simulink model "przyklad_mateusz"  (R2023a)
settings: Solver=ode1  StartTime=0.0  StopTime=inf  FixedStep=0.0001  RelTol=1e-3  EnableMultiTasking=on
undefined symbols (not defined in the file): DiscIntNeverNeededParam, sigbuilder_block
libraries: stm32f4xxblockslib x8, simulink x7, stm32blockslib x6, stmutilitieslib x3, stm32f7xxblockslib x3
(part 2 of 2)

== system przyklad_mateusz/obiekt/fuzzy/Fuzzy Type 2/nbM5 ==
  x : Inport
  Add : Sum  Inputs=+-
  Add1 : Sum  Inputs=-+
  Add2 : Sum  Inputs=+-
  Add3 : Sum  Inputs=-+
  Constant : Constant
  Constant1 : Constant
  Constant2 : Constant  Value=0
  Divide : Product  Inputs=*/
  Divide1 : Product  Inputs=*/
  Max : MinMax  Function=max  Inputs=2
  Min : MinMax  Inputs=2
  Switch : Switch  Criteria=u2 > Threshold  SaturateOnIntegerOverflow=off  InputSameDT=off
  Switch1 : Switch  Criteria=u2 > Threshold  SaturateOnIntegerOverflow=off  InputSameDT=off
  a : Constant  Value=-1.8
  b : Constant  Value=-1
  c : Constant  Value=-0.2
  Out1 : Outport
  wires:
  x/1 -> Add2/2, Add/1
  a/1 -> Add1/1, Add/2
  b/1 -> Add1/2, Add3/1
  c/1 -> Add2/1, Add3/2
  Add/1 -> Divide/1
  Divide1/1 -> Switch1/1
  Divide/1 -> Switch/1
  Add1/1 -> Switch/2, Divide/2
  Add2/1 -> Divide1/1
  Add3/1 -> Switch1/2, Divide1/2
  Constant/1 -> Switch/3
  Constant1/1 -> Switch1/3
  Switch/1 -> Min/1
  Switch1/1 -> Min/2
  Min/1 -> Max/2
  Constant2/1 -> Max/1
  Max/1 -> Out1/1

== system przyklad_mateusz/obiekt/fuzzy/Fuzzy Type 2/pbM2 ==
  x : Inport
  Add : Sum  Inputs=+-
  Add1 : Sum  Inputs=-+
  Add2 : Sum  Inputs=+-
  Add3 : Sum  Inputs=-+
  Constant : Constant
  Constant1 : Constant
  Constant2 : Constant  Value=0
  Divide : Product  Inputs=*/
  Divide1 : Product  Inputs=*/
  Max : MinMax  Function=max  Inputs=2
  Min : MinMax  Inputs=2
  Switch : Switch  Criteria=u2 > Threshold  SaturateOnIntegerOverflow=off  InputSameDT=off
  Switch1 : Switch  Criteria=u2 > Threshold  SaturateOnIntegerOverflow=off  InputSameDT=off
  a : Constant  Value=0
  b : Constant
  c : Constant  Value=2
  Out1 : Outport
  wires:
  Max/1 -> Out1/1
  Constant2/1 -> Max/1
  Min/1 -> Max/2
  Switch1/1 -> Min/2
  Switch/1 -> Min/1
  Constant1/1 -> Switch1/3
  Constant/1 -> Switch/3
  Add3/1 -> Divide1/2, Switch1/2
  Add2/1 -> Divide1/1
  Add1/1 -> Divide/2, Switch/2
  Divide/1 -> Switch/1
  Divide1/1 -> Switch1/1
  Add/1 -> Divide/1
  c/1 -> Add3/2, Add2/1
  b/1 -> Add3/1, Add1/2
  a/1 -> Add/2, Add1/1
  x/1 -> Add/1, Add2/2

== system przyklad_mateusz/obiekt/fuzzy/Fuzzy Type 2/pbM3 ==
  x : Inport
  Add : Sum  Inputs=+-
  Add1 : Sum  Inputs=-+
  Add2 : Sum  Inputs=+-
  Add3 : Sum  Inputs=-+
  Constant : Constant
  Constant1 : Constant
  Constant2 : Constant  Value=0
  Divide : Product  Inputs=*/
  Divide1 : Product  Inputs=*/
  Max : MinMax  Function=max  Inputs=2
  Min : MinMax  Inputs=2
  Switch : Switch  Criteria=u2 > Threshold  SaturateOnIntegerOverflow=off  InputSameDT=off
  Switch1 : Switch  Criteria=u2 > Threshold  SaturateOnIntegerOverflow=off  InputSameDT=off
  a : Constant  Value=0
  b : Constant
  c : Constant  Value=2
  Out1 : Outport
  wires:
  Max/1 -> Out1/1
  Constant2/1 -> Max/1
  Min/1 -> Max/2
  Switch1/1 -> Min/2
  Switch/1 -> Min/1
  Constant1/1 -> Switch1/3
  Constant/1 -> Switch/3
  Add3/1 -> Divide1/2, Switch1/2
  Add2/1 -> Divide1/1
  Add1/1 -> Divide/2, Switch/2
  Divide/1 -> Switch/1
  Divide1/1 -> Switch1/1
  Add/1 -> Divide/1
  c/1 -> Add3/2, Add2/1
  b/1 -> Add3/1, Add1/2
  a/1 -> Add/2, Add1/1
  x/1 -> Add/1, Add2/2

== system przyklad_mateusz/obiekt/fuzzy/Fuzzy Type 2/pbM4 ==
  x : Inport
  Add : Sum  Inputs=+-
  Add1 : Sum  Inputs=-+
  Add2 : Sum  Inputs=+-
  Add3 : Sum  Inputs=-+
  Constant : Constant
  Constant1 : Constant
  Constant2 : Constant  Value=0
  Divide : Product  Inputs=*/
  Divide1 : Product  Inputs=*/
  Max : MinMax  Function=max  Inputs=2
  Min : MinMax  Inputs=2
  Switch : Switch  Criteria=u2 > Threshold  SaturateOnIntegerOverflow=off  InputSameDT=off
  Switch1 : Switch  Criteria=u2 > Threshold  SaturateOnIntegerOverflow=off  InputSameDT=off
  a : Constant  Value=0.2
  b : Constant
  c : Constant  Value=1.8
  Out1 : Outport
  wires:
  x/1 -> Add2/2, Add/1
  a/1 -> Add1/1, Add/2
  b/1 -> Add1/2, Add3/1
  c/1 -> Add2/1, Add3/2
  Add/1 -> Divide/1
  Divide1/1 -> Switch1/1
  Divide/1 -> Switch/1
  Add1/1 -> Switch/2, Divide/2
  Add2/1 -> Divide1/1
  Add3/1 -> Switch1/2, Divide1/2
  Constant/1 -> Switch/3
  Constant1/1 -> Switch1/3
  Switch/1 -> Min/1
  Switch1/1 -> Min/2
  Min/1 -> Max/2
  Constant2/1 -> Max/1
  Max/1 -> Out1/1

== system przyklad_mateusz/obiekt/fuzzy/Fuzzy Type 2/pbM5 ==
  x : Inport
  Add : Sum  Inputs=+-
  Add1 : Sum  Inputs=-+
  Add2 : Sum  Inputs=+-
  Add3 : Sum  Inputs=-+
  Constant : Constant
  Constant1 : Constant
  Constant2 : Constant  Value=0
  Divide : Product  Inputs=*/
  Divide1 : Product  Inputs=*/
  Max : MinMax  Function=max  Inputs=2
  Min : MinMax  Inputs=2
  Switch : Switch  Criteria=u2 > Threshold  SaturateOnIntegerOverflow=off  InputSameDT=off
  Switch1 : Switch  Criteria=u2 > Threshold  SaturateOnIntegerOverflow=off  InputSameDT=off
  a : Constant  Value=0.2
  b : Constant
  c : Constant  Value=1.8
  Out1 : Outport
  wires:
  x/1 -> Add2/2, Add/1
  a/1 -> Add1/1, Add/2
  b/1 -> Add1/2, Add3/1
  c/1 -> Add2/1, Add3/2
  Add/1 -> Divide/1
  Divide1/1 -> Switch1/1
  Divide/1 -> Switch/1
  Add1/1 -> Switch/2, Divide/2
  Add2/1 -> Divide1/1
  Add3/1 -> Switch1/2, Divide1/2
  Constant/1 -> Switch/3
  Constant1/1 -> Switch1/3
  Switch/1 -> Min/1
  Switch1/1 -> Min/2
  Min/1 -> Max/2
  Constant2/1 -> Max/1
  Max/1 -> Out1/1

== system przyklad_mateusz/obiekt/fuzzy/Fuzzy Type 2/zeM2 ==
  x : Inport
  Add : Sum  Inputs=+-
  Add1 : Sum  Inputs=-+
  Add2 : Sum  Inputs=+-
  Add3 : Sum  Inputs=-+
  Constant : Constant
  Constant1 : Constant
  Constant2 : Constant  Value=0
  Divide : Product  Inputs=*/
  Divide1 : Product  Inputs=*/
  Max : MinMax  Function=max  Inputs=2
  Min : MinMax  Inputs=2
  Switch : Switch  Criteria=u2 > Threshold  SaturateOnIntegerOverflow=off  InputSameDT=off
  Switch1 : Switch  Criteria=u2 > Threshold  SaturateOnIntegerOverflow=off  InputSameDT=off
  a : Constant  Value=-1
  b : Constant  Value=0
  c : Constant
  Out1 : Outport
  wires:
  Max/1 -> Out1/1
  Constant2/1 -> Max/1
  Min/1 -> Max/2
  Switch1/1 -> Min/2
  Switch/1 -> Min/1
  Constant1/1 -> Switch1/3
  Constant/1 -> Switch/3
  Add3/1 -> Divide1/2, Switch1/2
  Add2/1 -> Divide1/1
  Add1/1 -> Divide/2, Switch/2
  Divide/1 -> Switch/1
  Divide1/1 -> Switch1/1
  Add/1 -> Divide/1
  c/1 -> Add3/2, Add2/1
  b/1 -> Add3/1, Add1/2
  a/1 -> Add/2, Add1/1
  x/1 -> Add/1, Add2/2

== system przyklad_mateusz/obiekt/fuzzy/Fuzzy Type 2/zeM3 ==
  x : Inport
  Add : Sum  Inputs=+-
  Add1 : Sum  Inputs=-+
  Add2 : Sum  Inputs=+-
  Add3 : Sum  Inputs=-+
  Constant : Constant
  Constant1 : Constant
  Constant2 : Constant  Value=0
  Divide : Product  Inputs=*/
  Divide1 : Product  Inputs=*/
  Max : MinMax  Function=max  Inputs=2
  Min : MinMax  Inputs=2
  Switch : Switch  Criteria=u2 > Threshold  SaturateOnIntegerOverflow=off  InputSameDT=off
  Switch1 : Switch  Criteria=u2 > Threshold  SaturateOnIntegerOverflow=off  InputSameDT=off
  a : Constant  Value=-1
  b : Constant  Value=0
  c : Constant
  Out1 : Outport
  wires:
  Max/1 -> Out1/1
  Constant2/1 -> Max/1
  Min/1 -> Max/2
  Switch1/1 -> Min/2
  Switch/1 -> Min/1
  Constant1/1 -> Switch1/3
  Constant/1 -> Switch/3
  Add3/1 -> Divide1/2, Switch1/2
  Add2/1 -> Divide1/1
  Add1/1 -> Divide/2, Switch/2
  Divide/1 -> Switch/1
  Divide1/1 -> Switch1/1
  Add/1 -> Divide/1
  c/1 -> Add3/2, Add2/1
  b/1 -> Add3/1, Add1/2
  a/1 -> Add/2, Add1/1
  x/1 -> Add/1, Add2/2

== system przyklad_mateusz/obiekt/fuzzy/Fuzzy Type 2/zeM4 ==
  x : Inport
  Add : Sum  Inputs=+-
  Add1 : Sum  Inputs=-+
  Add2 : Sum  Inputs=+-
  Add3 : Sum  Inputs=-+
  Constant : Constant
  Constant1 : Constant
  Constant2 : Constant  Value=0
  Divide : Product  Inputs=*/
  Divide1 : Product  Inputs=*/
  Max : MinMax  Function=max  Inputs=2
  Min : MinMax  Inputs=2
  Switch : Switch  Criteria=u2 > Threshold  SaturateOnIntegerOverflow=off  InputSameDT=off
  Switch1 : Switch  Criteria=u2 > Threshold  SaturateOnIntegerOverflow=off  InputSameDT=off
  a : Constant  Value=-0.8
  b : Constant  Value=0
  c : Constant  Value=0.8
  Out1 : Outport
  wires:
  x/1 -> Add2/2, Add/1
  a/1 -> Add1/1, Add/2
  b/1 -> Add1/2, Add3/1
  c/1 -> Add2/1, Add3/2
  Add/1 -> Divide/1
  Divide1/1 -> Switch1/1
  Divide/1 -> Switch/1
  Add1/1 -> Switch/2, Divide/2
  Add2/1 -> Divide1/1
  Add3/1 -> Switch1/2, Divide1/2
  Constant/1 -> Switch/3
  Constant1/1 -> Switch1/3
  Switch/1 -> Min/1
  Switch1/1 -> Min/2
  Min/1 -> Max/2
  Constant2/1 -> Max/1
  Max/1 -> Out1/1

== system przyklad_mateusz/obiekt/fuzzy/Fuzzy Type 2/zeM5 ==
  x : Inport
  Add : Sum  Inputs=+-
  Add1 : Sum  Inputs=-+
  Add2 : Sum  Inputs=+-
  Add3 : Sum  Inputs=-+
  Constant : Constant
  Constant1 : Constant
  Constant2 : Constant  Value=0
  Divide : Product  Inputs=*/
  Divide1 : Product  Inputs=*/
  Max : MinMax  Function=max  Inputs=2
  Min : MinMax  Inputs=2
  Switch : Switch  Criteria=u2 > Threshold  SaturateOnIntegerOverflow=off  InputSameDT=off
  Switch1 : Switch  Criteria=u2 > Threshold  SaturateOnIntegerOverflow=off  InputSameDT=off
  a : Constant  Value=-0.8
  b : Constant  Value=0
  c : Constant  Value=0.8
  Out1 : Outport
  wires:
  x/1 -> Add2/2, Add/1
  a/1 -> Add1/1, Add/2
  b/1 -> Add1/2, Add3/1
  c/1 -> Add2/1, Add3/2
  Add/1 -> Divide/1
  Divide1/1 -> Switch1/1
  Divide/1 -> Switch/1
  Add1/1 -> Switch/2, Divide/2
  Add2/1 -> Divide1/1
  Add3/1 -> Switch1/2, Divide1/2
  Constant/1 -> Switch/3
  Constant1/1 -> Switch1/3
  Switch/1 -> Min/1
  Switch1/1 -> Min/2
  Min/1 -> Max/2
  Constant2/1 -> Max/1
  Max/1 -> Out1/1

== system przyklad_mateusz/Subsystem1/Subsystem/Enkoder/zliczanie enkodera/If Action Subsystem ==
  Input : Inport
  Input2 : Inport  Port=2
  Action Port : ActionPort
  If : If  IfExpression=u1 == 0  ShowElse=off
  If Action Subsystem : Subsystem  TreatAsAtomicUnit=on
  Out1 : Outport
  wires:
  Input/1 -> If/1
  If/1 -> If Action Subsystem/Action
  Input2/1 -> If Action Subsystem/1(Input2)
  If Action Subsystem/1(Out1) -> Out1/1

== system przyklad_mateusz/Subsystem1/Subsystem/Enkoder/zliczanie enkodera/If Action Subsystem2 ==
  Input : Inport
  Input2 : Inport  Port=2
  Action Port : ActionPort
  If : If  IfExpression=u1 == 1  ShowElse=off
  If Action Subsystem : Subsystem  TreatAsAtomicUnit=on
  Out1 : Outport
  wires:
  If Action Subsystem/1(Out1) -> Out1/1
  Input2/1 -> If Action Subsystem/1(Input2)
  If/1 -> If Action Subsystem/Action
  Input/1 -> If/1

== system przyklad_mateusz/Subsystem1/Subsystem/Obiekt/Moj/nbM ==
  x : Inport
  Add : Sum  Inputs=+-
  Add1 : Sum  Inputs=-+
  Add2 : Sum  Inputs=+-
  Add3 : Sum  Inputs=-+
  Constant : Constant
  Constant1 : Constant
  Constant2 : Constant  Value=0
  Divide : Product  Inputs=*/
  Divide1 : Product  Inputs=*/
  Max : MinMax  Function=max  Inputs=2
  Min : MinMax  Inputs=2
  Switch : Switch  Criteria=u2 > Threshold  SaturateOnIntegerOverflow=off  InputSameDT=off
  Switch1 : Switch  Criteria=u2 > Threshold  SaturateOnIntegerOverflow=off  InputSameDT=off
  a : Constant  Value=-2
  b : Constant  Value=-1
  c : Constant  Value=0
  Out1 : Outport
  wires:
  x/1 -> Add2/2, Add/1
  a/1 -> Add1/1, Add/2
  b/1 -> Add1/2, Add3/1
  c/1 -> Add2/1, Add3/2
  Add/1 -> Divide/1
  Divide1/1 -> Switch1/1
  Divide/1 -> Switch/1
  Add1/1 -> Switch/2, Divide/2
  Add2/1 -> Divide1/1
  Add3/1 -> Switch1/2, Divide1/2
  Constant/1 -> Switch/3
  Constant1/1 -> Switch1/3
  Switch/1 -> Min/1
  Switch1/1 -> Min/2
  Min/1 -> Max/2
  Constant2/1 -> Max/1
  Max/1 -> Out1/1

== system przyklad_mateusz/Subsystem1/Subsystem/Obiekt/Moj/nbM1 ==
  x : Inport
  Add : Sum  Inputs=+-
  Add1 : Sum  Inputs=-+
  Add2 : Sum  Inputs=+-
  Add3 : Sum  Inputs=-+
  Constant : Constant
  Constant1 : Constant
  Constant2 : Constant  Value=0
  Divide : Product  Inputs=*/
  Divide1 : Product  Inputs=*/
  Max : MinMax  Function=max  Inputs=2
  Min : MinMax  Inputs=2
  Switch : Switch  Criteria=u2 > Threshold  SaturateOnIntegerOverflow=off  InputSameDT=off
  Switch1 : Switch  Criteria=u2 > Threshold  SaturateOnIntegerOverflow=off  InputSameDT=off
  a : Constant  Value=-2
  b : Constant  Value=-1
  c : Constant  Value=0
  Out1 : Outport
  wires:
  x/1 -> Add2/2, Add/1
  a/1 -> Add1/1, Add/2
  b/1 -> Add1/2, Add3/1
  c/1 -> Add2/1, Add3/2
  Add/1 -> Divide/1
  Divide1/1 -> Switch1/1
  Divide/1 -> Switch/1
  Add1/1 -> Switch/2, Divide/2
  Add2/1 -> Divide1/1
  Add3/1 -> Switch1/2, Divide1/2
  Constant/1 -> Switch/3
  Constant1/1 -> Switch1/3
  Switch/1 -> Min/1
  Switch1/1 -> Min/2
  Min/1 -> Max/2
  Constant2/1 -> Max/1
  Max/1 -> Out1/1

== system przyklad_mateusz/Subsystem1/Subsystem/Obiekt/Moj/pbM ==
  x : Inport
  Add : Sum  Inputs=+-
  Add1 : Sum  Inputs=-+
  Add2 : Sum  Inputs=+-
  Add3 : Sum  Inputs=-+
  Constant : Constant
  Constant1 : Constant
  Constant2 : Constant  Value=0
  Divide : Product  Inputs=*/
  Divide1 : Product  Inputs=*/
  Max : MinMax  Function=max  Inputs=2
  Min : MinMax  Inputs=2
  Switch : Switch  Criteria=u2 > Threshold  SaturateOnIntegerOverflow=off  InputSameDT=off
  Switch1 : Switch  Criteria=u2 > Threshold  SaturateOnIntegerOverflow=off  InputSameDT=off
  a : Constant  Value=0
  b : Constant
  c : Constant  Value=2
  Out1 : Outport
  wires:
  x/1 -> Add2/2, Add/1
  a/1 -> Add1/1, Add/2
  b/1 -> Add1/2, Add3/1
  c/1 -> Add2/1, Add3/2
  Add/1 -> Divide/1
  Divide1/1 -> Switch1/1
  Divide/1 -> Switch/1
  Add1/1 -> Switch/2, Divide/2
  Add2/1 -> Divide1/1
  Add3/1 -> Switch1/2, Divide1/2
  Constant/1 -> Switch/3
  Constant1/1 -> Switch1/3
  Switch/1 -> Min/1
  Switch1/1 -> Min/2
  Min/1 -> Max/2
  Constant2/1 -> Max/1
  Max/1 -> Out1/1

== system przyklad_mateusz/Subsystem1/Subsystem/Obiekt/Moj/pbM1 ==
  x : Inport
  Add : Sum  Inputs=+-
  Add1 : Sum  Inputs=-+
  Add2 : Sum  Inputs=+-
  Add3 : Sum  Inputs=-+
  Constant : Constant
  Constant1 : Constant
  Constant2 : Constant  Value=0
  Divide : Product  Inputs=*/
  Divide1 : Product  Inputs=*/
  Max : MinMax  Function=max  Inputs=2
  Min : MinMax  Inputs=2
  Switch : Switch  Criteria=u2 > Threshold  SaturateOnIntegerOverflow=off  InputSameDT=off
  Switch1 : Switch  Criteria=u2 > Threshold  SaturateOnIntegerOverflow=off  InputSameDT=off
  a : Constant  Value=0
  b : Constant
  c : Constant  Value=2
  Out1 : Outport
  wires:
  x/1 -> Add2/2, Add/1
  a/1 -> Add1/1, Add/2
  b/1 -> Add1/2, Add3/1
  c/1 -> Add2/1, Add3/2
  Add/1 -> Divide/1
  Divide1/1 -> Switch1/1
  Divide/1 -> Switch/1
  Add1/1 -> Switch/2, Divide/2
  Add2/1 -> Divide1/1
  Add3/1 -> Switch1/2, Divide1/2
  Constant/1 -> Switch/3
  Constant1/1 -> Switch1/3
  Switch/1 -> Min/1
  Switch1/1 -> Min/2
  Min/1 -> Max/2
  Constant2/1 -> Max/1
  Max/1 -> Out1/1

== system przyklad_mateusz/Subsystem1/Subsystem/Obiekt/Moj/zeM ==
  x : Inport
  Add : Sum  Inputs=+-
  Add1 : Sum  Inputs=-+
  Add2 : Sum  Inputs=+-
  Add3 : Sum  Inputs=-+
  Constant : Constant
  Constant1 : Constant
  Constant2 : Constant  Value=0
  Divide : Product  Inputs=*/
  Divide1 : Product  Inputs=*/
  Max : MinMax  Function=max  Inputs=2
  Min : MinMax  Inputs=2
  Switch : Switch  Criteria=u2 > Threshold  SaturateOnIntegerOverflow=off  InputSameDT=off
  Switch1 : Switch  Criteria=u2 > Threshold  SaturateOnIntegerOverflow=off  InputSameDT=off
  a : Constant  Value=-1
  b : Constant  Value=0
  c : Constant
  Out1 : Outport
  wires:
  x/1 -> Add2/2, Add/1
  a/1 -> Add1/1, Add/2
  b/1 -> Add1/2, Add3/1
  c/1 -> Add2/1, Add3/2
  Add/1 -> Divide/1
  Divide1/1 -> Switch1/1
  Divide/1 -> Switch/1
  Add1/1 -> Switch/2, Divide/2
  Add2/1 -> Divide1/1
  Add3/1 -> Switch1/2, Divide1/2
  Constant/1 -> Switch/3
  Constant1/1 -> Switch1/3
  Switch/1 -> Min/1
  Switch1/1 -> Min/2
  Min/1 -> Max/2
  Constant2/1 -> Max/1
  Max/1 -> Out1/1

== system przyklad_mateusz/Subsystem1/Subsystem/Obiekt/Moj/zeM1 ==
  x : Inport
  Add : Sum  Inputs=+-
  Add1 : Sum  Inputs=-+
  Add2 : Sum  Inputs=+-
  Add3 : Sum  Inputs=-+
  Constant : Constant
  Constant1 : Constant
  Constant2 : Constant  Value=0
  Divide : Product  Inputs=*/
  Divide1 : Product  Inputs=*/
  Max : MinMax  Function=max  Inputs=2
  Min : MinMax  Inputs=2
  Switch : Switch  Criteria=u2 > Threshold  SaturateOnIntegerOverflow=off  InputSameDT=off
  Switch1 : Switch  Criteria=u2 > Threshold  SaturateOnIntegerOverflow=off  InputSameDT=off
  a : Constant  Value=-1
  b : Constant  Value=0
  c : Constant
  Out1 : Outport
  wires:
  x/1 -> Add2/2, Add/1
  a/1 -> Add1/1, Add/2
  b/1 -> Add1/2, Add3/1
  c/1 -> Add2/1, Add3/2
  Add/1 -> Divide/1
  Divide1/1 -> Switch1/1
  Divide/1 -> Switch/1
  Add1/1 -> Switch/2, Divide/2
  Add2/1 -> Divide1/1
  Add3/1 -> Switch1/2, Divide1/2
  Constant/1 -> Switch/3
  Constant1/1 -> Switch1/3
  Switch/1 -> Min/1
  Switch1/1 -> Min/2
  Min/1 -> Max/2
  Constant2/1 -> Max/1
  Max/1 -> Out1/1

== system przyklad_mateusz/Subsystem1/Subsystem/regulator/fuzzy/nbM ==
  x : Inport
  Add : Sum  Inputs=+-
  Add1 : Sum  Inputs=-+
  Add2 : Sum  Inputs=+-
  Add3 : Sum  Inputs=-+
  Constant : Constant
  Constant1 : Constant
  Constant2 : Constant  Value=0
  Divide : Product  Inputs=*/
  Divide1 : Product  Inputs=*/
  Max : MinMax  Function=max  Inputs=2
  Min : MinMax  Inputs=2
  Switch : Switch  Criteria=u2 > Threshold  SaturateOnIntegerOverflow=off  InputSameDT=off
  Switch1 : Switch  Criteria=u2 > Threshold  SaturateOnIntegerOverflow=off  InputSameDT=off
  a : Constant  Value=-2
  b : Constant  Value=-1
  c : Constant  Value=0
  Out1 : Outport
  wires:
  x/1 -> Add2/2, Add/1
  a/1 -> Add1/1, Add/2
  b/1 -> Add1/2, Add3/1
  c/1 -> Add2/1, Add3/2
  Add/1 -> Divide/1
  Divide1/1 -> Switch1/1
  Divide/1 -> Switch/1
  Add1/1 -> Switch/2, Divide/2
  Add2/1 -> Divide1/1
  Add3/1 -> Switch1/2, Divide1/2
  Constant/1 -> Switch/3
  Constant1/1 -> Switch1/3
  Switch/1 -> Min/1
  Switch1/1 -> Min/2
  Min/1 -> Max/2
  Constant2/1 -> Max/1
  Max/1 -> Out1/1

== system przyklad_mateusz/Subsystem1/Subsystem/regulator/fuzzy/nbM1 ==
  x : Inport
  Add : Sum  Inputs=+-
  Add1 : Sum  Inputs=-+
  Add2 : Sum  Inputs=+-
  Add3 : Sum  Inputs=-+
  Constant : Constant
  Constant1 : Constant
  Constant2 : Constant  Value=0
  Divide : Product  Inputs=*/
  Divide1 : Product  Inputs=*/
  Max : MinMax  Function=max  Inputs=2
  Min : MinMax  Inputs=2
  Switch : Switch  Criteria=u2 > Threshold  SaturateOnIntegerOverflow=off  InputSameDT=off
  Switch1 : Switch  Criteria=u2 > Threshold  SaturateOnIntegerOverflow=off  InputSameDT=off
  a : Constant  Value=-2
  b : Constant  Value=-1
  c : Constant  Value=0
  Out1 : Outport
  wires:
  x/1 -> Add2/2, Add/1
  a/1 -> Add1/1, Add/2
  b/1 -> Add1/2, Add3/1
  c/1 -> Add2/1, Add3/2
  Add/1 -> Divide/1
  Divide1/1 -> Switch1/1
  Divide/1 -> Switch/1
  Add1/1 -> Switch/2, Divide/2
  Add2/1 -> Divide1/1
  Add3/1 -> Switch1/2, Divide1/2
  Constant/1 -> Switch/3
  Constant1/1 -> Switch1/3
  Switch/1 -> Min/1
  Switch1/1 -> Min/2
  Min/1 -> Max/2
  Constant2/1 -> Max/1
  Max/1 -> Out1/1

== system przyklad_mateusz/Subsystem1/Subsystem/regulator/fuzzy/pbM ==
  x : Inport
  Add : Sum  Inputs=+-
  Add1 : Sum  Inputs=-+
  Add2 : Sum  Inputs=+-
  Add3 : Sum  Inputs=-+
  Constant : Constant
  Constant1 : Constant
  Constant2 : Constant  Value=0
  Divide : Product  Inputs=*/
  Divide1 : Product  Inputs=*/
  Max : MinMax  Function=max  Inputs=2
  Min : MinMax  Inputs=2
  Switch : Switch  Criteria=u2 > Threshold  SaturateOnIntegerOverflow=off  InputSameDT=off
  Switch1 : Switch  Criteria=u2 > Threshold  SaturateOnIntegerOverflow=off  InputSameDT=off
  a : Constant  Value=0
  b : Constant
  c : Constant  Value=2
  Out1 : Outport
  wires:
  x/1 -> Add2/2, Add/1
  a/1 -> Add1/1, Add/2
  b/1 -> Add1/2, Add3/1
  c/1 -> Add2/1, Add3/2
  Add/1 -> Divide/1
  Divide1/1 -> Switch1/1
  Divide/1 -> Switch/1
  Add1/1 -> Switch/2, Divide/2
  Add2/1 -> Divide1/1
  Add3/1 -> Switch1/2, Divide1/2
  Constant/1 -> Switch/3
  Constant1/1 -> Switch1/3
  Switch/1 -> Min/1
  Switch1/1 -> Min/2
  Min/1 -> Max/2
  Constant2/1 -> Max/1
  Max/1 -> Out1/1

== system przyklad_mateusz/Subsystem1/Subsystem/regulator/fuzzy/pbM1 ==
  x : Inport
  Add : Sum  Inputs=+-
  Add1 : Sum  Inputs=-+
  Add2 : Sum  Inputs=+-
  Add3 : Sum  Inputs=-+
  Constant : Constant
  Constant1 : Constant
  Constant2 : Constant  Value=0
  Divide : Product  Inputs=*/
  Divide1 : Product  Inputs=*/
  Max : MinMax  Function=max  Inputs=2
  Min : MinMax  Inputs=2
  Switch : Switch  Criteria=u2 > Threshold  SaturateOnIntegerOverflow=off  InputSameDT=off
  Switch1 : Switch  Criteria=u2 > Threshold  SaturateOnIntegerOverflow=off  InputSameDT=off
  a : Constant  Value=0
  b : Constant
  c : Constant  Value=2
  Out1 : Outport
  wires:
  x/1 -> Add2/2, Add/1
  a/1 -> Add1/1, Add/2
  b/1 -> Add1/2, Add3/1
  c/1 -> Add2/1, Add3/2
  Add/1 -> Divide/1
  Divide1/1 -> Switch1/1
  Divide/1 -> Switch/1
  Add1/1 -> Switch/2, Divide/2
  Add2/1 -> Divide1/1
  Add3/1 -> Switch1/2, Divide1/2
  Constant/1 -> Switch/3
  Constant1/1 -> Switch1/3
  Switch/1 -> Min/1
  Switch1/1 -> Min/2
  Min/1 -> Max/2
  Constant2/1 -> Max/1
  Max/1 -> Out1/1

== system przyklad_mateusz/Subsystem1/Subsystem/regulator/fuzzy/zeM ==
  x : Inport
  Add : Sum  Inputs=+-
  Add1 : Sum  Inputs=-+
  Add2 : Sum  Inputs=+-
  Add3 : Sum  Inputs=-+
  Constant : Constant
  Constant1 : Constant
  Constant2 : Constant  Value=0
  Divide : Product  Inputs=*/
  Divide1 : Product  Inputs=*/
  Max : MinMax  Function=max  Inputs=2
  Min : MinMax  Inputs=2
  Switch : Switch  Criteria=u2 > Threshold  SaturateOnIntegerOverflow=off  InputSameDT=off
  Switch1 : Switch  Criteria=u2 > Threshold  SaturateOnIntegerOverflow=off  InputSameDT=off
  a : Constant  Value=-1
  b : Constant  Value=0
  c : Constant
  Out1 : Outport
  wires:
  x/1 -> Add2/2, Add/1
  a/1 -> Add1/1, Add/2
  b/1 -> Add1/2, Add3/1
  c/1 -> Add2/1, Add3/2
  Add/1 -> Divide/1
  Divide1/1 -> Switch1/1
  Divide/1 -> Switch/1
  Add1/1 -> Switch/2, Divide/2
  Add2/1 -> Divide1/1
  Add3/1 -> Switch1/2, Divide1/2
  Constant/1 -> Switch/3
  Constant1/1 -> Switch1/3
  Switch/1 -> Min/1
  Switch1/1 -> Min/2
  Min/1 -> Max/2
  Constant2/1 -> Max/1
  Max/1 -> Out1/1

== system przyklad_mateusz/Subsystem1/Subsystem/regulator/fuzzy/zeM1 ==
  x : Inport
  Add : Sum  Inputs=+-
  Add1 : Sum  Inputs=-+
  Add2 : Sum  Inputs=+-
  Add3 : Sum  Inputs=-+
  Constant : Constant
  Constant1 : Constant
  Constant2 : Constant  Value=0
  Divide : Product  Inputs=*/
  Divide1 : Product  Inputs=*/
  Max : MinMax  Function=max  Inputs=2
  Min : MinMax  Inputs=2
  Switch : Switch  Criteria=u2 > Threshold  SaturateOnIntegerOverflow=off  InputSameDT=off
  Switch1 : Switch  Criteria=u2 > Threshold  SaturateOnIntegerOverflow=off  InputSameDT=off
  a : Constant  Value=-1
  b : Constant  Value=0
  c : Constant
  Out1 : Outport
  wires:
  x/1 -> Add2/2, Add/1
  a/1 -> Add1/1, Add/2
  b/1 -> Add1/2, Add3/1
  c/1 -> Add2/1, Add3/2
  Add/1 -> Divide/1
  Divide1/1 -> Switch1/1
  Divide/1 -> Switch/1
  Add1/1 -> Switch/2, Divide/2
  Add2/1 -> Divide1/1
  Add3/1 -> Switch1/2, Divide1/2
  Constant/1 -> Switch/3
  Constant1/1 -> Switch1/3
  Switch/1 -> Min/1
  Switch1/1 -> Min/2
  Min/1 -> Max/2
  Constant2/1 -> Max/1
  Max/1 -> Out1/1

== system przyklad_mateusz/Subsystem1/Subsystem/Enkoder/zliczanie enkodera/If Action Subsystem/If Action Subsystem ==
  Input2 : Inport
  Action Port : ActionPort
  Add : Sum
  Memory : Memory  InheritSampleTime=on
  Out1 : Outport
  wires:
  Add/1 -> Out1/1, Memory/1
  Input2/1 -> Add/1
  Memory/1 -> Add/2

== system przyklad_mateusz/Subsystem1/Subsystem/Enkoder/zliczanie enkodera/If Action Subsystem2/If Action Subsystem ==
  Input2 : Inport
  Action Port : ActionPort
  Add : Sum
  Memory : Memory  InheritSampleTime=on
  Out1 : Outport
  wires:
  Memory/1 -> Add/2
  Input2/1 -> Add/1
  Add/1 -> Out1/1, Memory/1
